simulink model "vuum_wab_4x1_mux"  (R2012b)
settings: Solver=ode45  StartTime=0.0  StopTime=10.0  RelTol=1e-3
libraries: xbsIndex_r4 x210
settings Model: Creator=rng  LastModifiedBy=rng

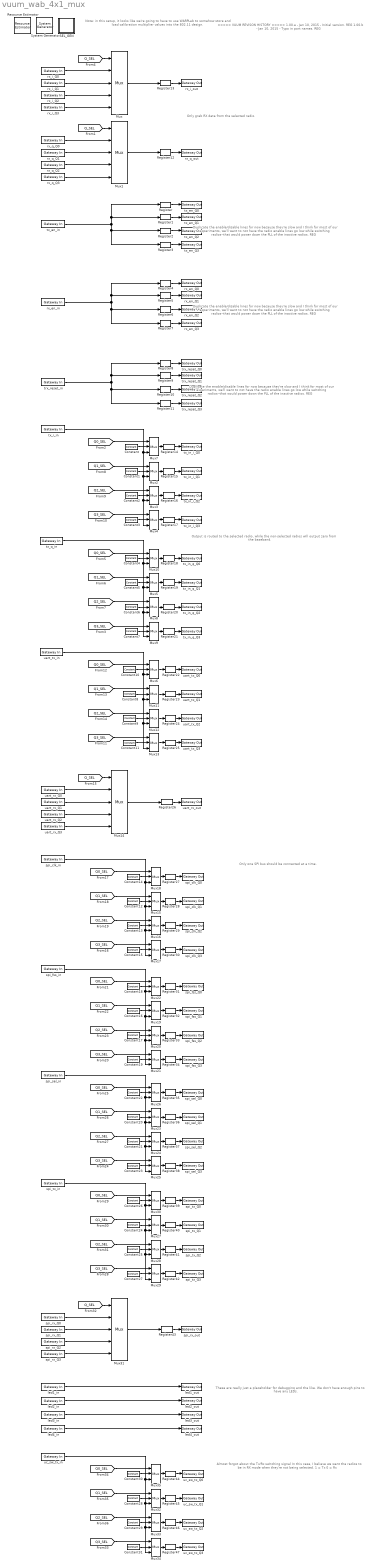
== system vuum_wab_4x1_mux ==
  note: Almost forgot about the Tx/Rx switching signal
      | In this case, I believe we want the radios to be
      | in RX mode when they're not being selected.
      | 1 = Tx
      | 0 = Rx
  note: ===== VUUM REVISON HISTORY =====
      | 1.00.a - Jan 10, 2015 - Initial version. REG
      | 1.00.b - Jan 10, 2015 - Typo in port names. REG
  note: These are really just a placeholder for debugging
      | and the like. We don't have enough pins to have any LEDs.
  note: Only one SPI bus should be connected at a time.
  note: Output is routed to the selected radio, while the
      | non-selected radios will output zero from the
      | baseband.
  note: Duplicate the enable/disable lines for now
      | because they're slow and I think for most
      | of our experiments, we'll want to not have
      | the radio enable lines go low while switching
      | radios--that would power down the PLL of the
      | inactive radios. REG
  note: Only grab RX data from the selected radio.
  note: Note: in this setup, it looks like we're going to have to use WARPLab
      | to somehow store and load calibration multiplier values into the 802.11
      | design.
  note: Duplicate the enable/disable lines for now
      | because they're slow and I think for most
      | of our experiments, we'll want to not have
      | the radio enable lines go low while switching
      | radios--that would power down the PLL of the
      | inactive radios. REG
  note: Duplicate the enable/disable lines for now
      | because they're slow and I think for most
      | of our experiments, we'll want to not have
      | the radio enable lines go low while switching
      | radios--that would power down the PLL of the
      | inactive radios. REG
  " System Generator" : xbsIndex_r4/ System Generator  Tag=genX  xilinxfamily=virtex6  part=xc6vlx240t  speed=-2  package=ff1156  synthesis_tool=XST  clock_wrapper=Clock Enables  directory=./vuum_wab_4x1_mux  proj_type=Project Navigator  Synth_file=XST Defaults  Impl_file=ISE Defaults  testbench=off  simulink_period=1  sysclk_period=10  dcm_input_clock_period=100  incr_netlist=off  trim_vbits=Everywhere in SubSystem  dbl_ovrd=According to Block Masks  core_generation=According to Block Masks  run_coregen=off  deprecated_control=off  eval_field=0  block_type=sysgen
      settings: block_version=10.1.3
  Constant{,1..7} (8 alike) : xbsIndex_r4/Constant  const=0  gui_display_data_type=Fixed-point  arith_type=Signed (2's comp)  n_bits=12  bin_pt=11  preci_type=Single  exp_width=8  frac_width=24  explicit_period=off  period=1  equ=P=C  opselect=C  inp2=PCIN>>17  opr=+  inp1=P  carry=CIN  dbl_ovrd=off  block_type=constant
  Constant{8..31} (24 alike) : xbsIndex_r4/Constant  const=0  gui_display_data_type=Boolean  arith_type=Boolean  n_bits=12  bin_pt=11  preci_type=Single  exp_width=8  frac_width=24  explicit_period=off  period=1  equ=P=C  opselect=C  inp2=PCIN>>17  opr=+  inp1=P  carry=CIN  dbl_ovrd=off  block_type=constant
  Mux{,1,14,31} (4 alike) : xbsIndex_r4/Mux  inputs=4  en=off  latency=0  precision=Full  arith_type=Unsigned  n_bits=16  bin_pt=14  quantization=Truncate  overflow=Wrap  dbl_ovrd=off  block_type=mux
  Mux{2..13,15..30,32..35} (32 alike) : xbsIndex_r4/Mux  inputs=2  en=off  latency=0  precision=Full  arith_type=Unsigned  n_bits=16  bin_pt=14  quantization=Truncate  overflow=Wrap  dbl_ovrd=off  block_type=mux
  Register{,1..47} (48 alike) : xbsIndex_r4/Register  init=0  rst=off  en=off  dbl_ovrd=off  block_type=register
  Resource Estimator : xbsIndex_r4/Resource Estimator  Tag=resEstTag  Slices=3628  FFs=4465  BRAMs=0  LUTs=6136  IOBs=365  EBMs=48  TBUFs=0  xl_use_estimator_area=off  est_options=Post Map  xl_estimator_area=[3628 4465 0 6136 365 48 0]  block_type=resource_estimator
      settings: AttributesFormatString=Resource\nEstimator  block_version=10.1.3
  SEL_GEN : Subsystem
  led1_in : xbsIndex_r4/Gateway In  gui_display_data_type=Boolean  arith_type=Boolean  n_bits=12  bin_pt=11  preci_type=Single  exp_width=8  frac_width=24  quantization="Round  (unbiased: +/- Inf)"  overflow=Saturate  period=1  dbl_ovrd=off  timing_constraint=None  locs_specified=off  LOCs={}  UseAsADC=off  ADCChannel='1'  inherit_from_input=off  hdl_port=on  block_type=gatewayin
  led1_out : xbsIndex_r4/Gateway Out  inherit_from_input=off  hdl_port=on  timing_constraint=None  locs_specified=off  LOCs={}  UseAsDAC=off  DACChannel='1'  block_type=gatewayout
  led2_in : xbsIndex_r4/Gateway In  gui_display_data_type=Boolean  arith_type=Boolean  n_bits=12  bin_pt=11  preci_type=Single  exp_width=8  frac_width=24  quantization="Round  (unbiased: +/- Inf)"  overflow=Saturate  period=1  dbl_ovrd=off  timing_constraint=None  locs_specified=off  LOCs={}  UseAsADC=off  ADCChannel='1'  inherit_from_input=off  hdl_port=on  block_type=gatewayin
  led2_out : xbsIndex_r4/Gateway Out  inherit_from_input=off  hdl_port=on  timing_constraint=None  locs_specified=off  LOCs={}  UseAsDAC=off  DACChannel='1'  block_type=gatewayout
  led3_in : xbsIndex_r4/Gateway In  gui_display_data_type=Boolean  arith_type=Boolean  n_bits=12  bin_pt=11  preci_type=Single  exp_width=8  frac_width=24  quantization="Round  (unbiased: +/- Inf)"  overflow=Saturate  period=1  dbl_ovrd=off  timing_constraint=None  locs_specified=off  LOCs={}  UseAsADC=off  ADCChannel='1'  inherit_from_input=off  hdl_port=on  block_type=gatewayin
  led3_out : xbsIndex_r4/Gateway Out  inherit_from_input=off  hdl_port=on  timing_constraint=None  locs_specified=off  LOCs={}  UseAsDAC=off  DACChannel='1'  block_type=gatewayout
  led4_in : xbsIndex_r4/Gateway In  gui_display_data_type=Boolean  arith_type=Boolean  n_bits=12  bin_pt=11  preci_type=Single  exp_width=8  frac_width=24  quantization="Round  (unbiased: +/- Inf)"  overflow=Saturate  period=1  dbl_ovrd=off  timing_constraint=None  locs_specified=off  LOCs={}  UseAsADC=off  ADCChannel='1'  inherit_from_input=off  hdl_port=on  block_type=gatewayin
  led4_out : xbsIndex_r4/Gateway Out  inherit_from_input=off  hdl_port=on  timing_constraint=None  locs_specified=off  LOCs={}  UseAsDAC=off  DACChannel='1'  block_type=gatewayout
  rx_en_Q{0..3} (4 alike) : xbsIndex_r4/Gateway Out  inherit_from_input=off  hdl_port=on  timing_constraint=None  locs_specified=off  LOCs={}  UseAsDAC=off  DACChannel='1'  block_type=gatewayout
  rx_en_in : xbsIndex_r4/Gateway In  gui_display_data_type=Boolean  arith_type=Boolean  n_bits=12  bin_pt=11  preci_type=Single  exp_width=8  frac_width=24  quantization="Round  (unbiased: +/- Inf)"  overflow=Saturate  period=1  dbl_ovrd=off  timing_constraint=None  locs_specified=off  LOCs={}  UseAsADC=off  ADCChannel='1'  inherit_from_input=off  hdl_port=on  block_type=gatewayin
  rx_i_Q{0..3} (4 alike) : xbsIndex_r4/Gateway In  gui_display_data_type=Fixed-point  arith_type="Signed  (2's comp)"  n_bits=12  bin_pt=11  preci_type=Single  exp_width=8  frac_width=24  quantization="Round  (unbiased: +/- Inf)"  overflow=Saturate  period=1  dbl_ovrd=off  timing_constraint=None  locs_specified=off  LOCs={}  UseAsADC=off  ADCChannel='1'  inherit_from_input=off  hdl_port=on  block_type=gatewayin
  rx_i_out : xbsIndex_r4/Gateway Out  inherit_from_input=off  hdl_port=on  timing_constraint=None  locs_specified=off  LOCs={}  UseAsDAC=off  DACChannel='1'  block_type=gatewayout
  rx_q_Q{0..3} (4 alike) : xbsIndex_r4/Gateway In  gui_display_data_type=Fixed-point  arith_type="Signed  (2's comp)"  n_bits=12  bin_pt=11  preci_type=Single  exp_width=8  frac_width=24  quantization="Round  (unbiased: +/- Inf)"  overflow=Saturate  period=1  dbl_ovrd=off  timing_constraint=None  locs_specified=off  LOCs={}  UseAsADC=off  ADCChannel='1'  inherit_from_input=off  hdl_port=on  block_type=gatewayin
  rx_q_out : xbsIndex_r4/Gateway Out  inherit_from_input=off  hdl_port=on  timing_constraint=None  locs_specified=off  LOCs={}  UseAsDAC=off  DACChannel='1'  block_type=gatewayout
  spi_clk_Q{0..3} (4 alike) : xbsIndex_r4/Gateway Out  inherit_from_input=off  hdl_port=on  timing_constraint=None  locs_specified=off  LOCs={}  UseAsDAC=off  DACChannel='1'  block_type=gatewayout
  spi_clk_in : xbsIndex_r4/Gateway In  gui_display_data_type=Boolean  arith_type=Boolean  n_bits=12  bin_pt=11  preci_type=Single  exp_width=8  frac_width=24  quantization="Round  (unbiased: +/- Inf)"  overflow=Saturate  period=1  dbl_ovrd=off  timing_constraint=None  locs_specified=off  LOCs={}  UseAsADC=off  ADCChannel='1'  inherit_from_input=off  hdl_port=on  block_type=gatewayin
  spi_fss_Q{0..3} (4 alike) : xbsIndex_r4/Gateway Out  inherit_from_input=off  hdl_port=on  timing_constraint=None  locs_specified=off  LOCs={}  UseAsDAC=off  DACChannel='1'  block_type=gatewayout
  spi_fss_in : xbsIndex_r4/Gateway In  gui_display_data_type=Boolean  arith_type=Boolean  n_bits=12  bin_pt=11  preci_type=Single  exp_width=8  frac_width=24  quantization="Round  (unbiased: +/- Inf)"  overflow=Saturate  period=1  dbl_ovrd=off  timing_constraint=None  locs_specified=off  LOCs={}  UseAsADC=off  ADCChannel='1'  inherit_from_input=off  hdl_port=on  block_type=gatewayin
  spi_rx_Q{0..3} (4 alike) : xbsIndex_r4/Gateway In  gui_display_data_type=Boolean  arith_type=Boolean  n_bits=12  bin_pt=11  preci_type=Single  exp_width=8  frac_width=24  quantization="Round  (unbiased: +/- Inf)"  overflow=Saturate  period=1  dbl_ovrd=off  timing_constraint=None  locs_specified=off  LOCs={}  UseAsADC=off  ADCChannel='1'  inherit_from_input=off  hdl_port=on  block_type=gatewayin
  spi_rx_out : xbsIndex_r4/Gateway Out  inherit_from_input=off  hdl_port=on  timing_constraint=None  locs_specified=off  LOCs={}  UseAsDAC=off  DACChannel='1'  block_type=gatewayout
  spi_sel_Q{0..3} (4 alike) : xbsIndex_r4/Gateway Out  inherit_from_input=off  hdl_port=on  timing_constraint=None  locs_specified=off  LOCs={}  UseAsDAC=off  DACChannel='1'  block_type=gatewayout
  spi_sel_in : xbsIndex_r4/Gateway In  gui_display_data_type=Boolean  arith_type=Boolean  n_bits=12  bin_pt=11  preci_type=Single  exp_width=8  frac_width=24  quantization="Round  (unbiased: +/- Inf)"  overflow=Saturate  period=1  dbl_ovrd=off  timing_constraint=None  locs_specified=off  LOCs={}  UseAsADC=off  ADCChannel='1'  inherit_from_input=off  hdl_port=on  block_type=gatewayin
  spi_tx_Q{0..3} (4 alike) : xbsIndex_r4/Gateway Out  inherit_from_input=off  hdl_port=on  timing_constraint=None  locs_specified=off  LOCs={}  UseAsDAC=off  DACChannel='1'  block_type=gatewayout
  spi_tx_in : xbsIndex_r4/Gateway In  gui_display_data_type=Boolean  arith_type=Boolean  n_bits=12  bin_pt=11  preci_type=Single  exp_width=8  frac_width=24  quantization="Round  (unbiased: +/- Inf)"  overflow=Saturate  period=1  dbl_ovrd=off  timing_constraint=None  locs_specified=off  LOCs={}  UseAsADC=off  ADCChannel='1'  inherit_from_input=off  hdl_port=on  block_type=gatewayin
  trx_reset_Q{0..3} (4 alike) : xbsIndex_r4/Gateway Out  inherit_from_input=off  hdl_port=on  timing_constraint=None  locs_specified=off  LOCs={}  UseAsDAC=off  DACChannel='1'  block_type=gatewayout
  trx_reset_in : xbsIndex_r4/Gateway In  gui_display_data_type=Boolean  arith_type=Boolean  n_bits=12  bin_pt=11  preci_type=Single  exp_width=8  frac_width=24  quantization="Round  (unbiased: +/- Inf)"  overflow=Saturate  period=1  dbl_ovrd=off  timing_constraint=None  locs_specified=off  LOCs={}  UseAsADC=off  ADCChannel='1'  inherit_from_input=off  hdl_port=on  block_type=gatewayin
  tx_en_Q{0..3} (4 alike) : xbsIndex_r4/Gateway Out  inherit_from_input=off  hdl_port=on  timing_constraint=None  locs_specified=off  LOCs={}  UseAsDAC=off  DACChannel='1'  block_type=gatewayout
  tx_en_in : xbsIndex_r4/Gateway In  gui_display_data_type=Boolean  arith_type=Boolean  n_bits=12  bin_pt=11  preci_type=Single  exp_width=8  frac_width=24  quantization="Round  (unbiased: +/- Inf)"  overflow=Saturate  period=1  dbl_ovrd=off  timing_constraint=None  locs_specified=off  LOCs={}  UseAsADC=off  ADCChannel='1'  inherit_from_input=off  hdl_port=on  block_type=gatewayin
  tx_i_in : xbsIndex_r4/Gateway In  gui_display_data_type=Fixed-point  arith_type="Signed  (2's comp)"  n_bits=12  bin_pt=11  preci_type=Single  exp_width=8  frac_width=24  quantization="Round  (unbiased: +/- Inf)"  overflow=Saturate  period=1  dbl_ovrd=off  timing_constraint=None  locs_specified=off  LOCs={}  UseAsADC=off  ADCChannel='1'  inherit_from_input=off  hdl_port=on  block_type=gatewayin
  tx_in_i_Q{0..3} (4 alike) : xbsIndex_r4/Gateway Out  inherit_from_input=off  hdl_port=on  timing_constraint=None  locs_specified=off  LOCs={}  UseAsDAC=off  DACChannel='1'  block_type=gatewayout
  tx_in_q_Q{0..3} (4 alike) : xbsIndex_r4/Gateway Out  inherit_from_input=off  hdl_port=on  timing_constraint=None  locs_specified=off  LOCs={}  UseAsDAC=off  DACChannel='1'  block_type=gatewayout
  tx_q_in : xbsIndex_r4/Gateway In  gui_display_data_type=Fixed-point  arith_type="Signed  (2's comp)"  n_bits=12  bin_pt=11  preci_type=Single  exp_width=8  frac_width=24  quantization="Round  (unbiased: +/- Inf)"  overflow=Saturate  period=1  dbl_ovrd=off  timing_constraint=None  locs_specified=off  LOCs={}  UseAsADC=off  ADCChannel='1'  inherit_from_input=off  hdl_port=on  block_type=gatewayin
  uart_rx_Q{0..3} (4 alike) : xbsIndex_r4/Gateway In  gui_display_data_type=Boolean  arith_type=Boolean  n_bits=12  bin_pt=11  preci_type=Single  exp_width=8  frac_width=24  quantization="Round  (unbiased: +/- Inf)"  overflow=Saturate  period=1  dbl_ovrd=off  timing_constraint=None  locs_specified=off  LOCs={}  UseAsADC=off  ADCChannel='1'  inherit_from_input=off  hdl_port=on  block_type=gatewayin
  uart_rx_out : xbsIndex_r4/Gateway Out  inherit_from_input=off  hdl_port=on  timing_constraint=None  locs_specified=off  LOCs={}  UseAsDAC=off  DACChannel='1'  block_type=gatewayout
  uart_tx_Q{0..3} (4 alike) : xbsIndex_r4/Gateway Out  inherit_from_input=off  hdl_port=on  timing_constraint=None  locs_specified=off  LOCs={}  UseAsDAC=off  DACChannel='1'  block_type=gatewayout
  uart_tx_in : xbsIndex_r4/Gateway In  gui_display_data_type=Boolean  arith_type=Boolean  n_bits=12  bin_pt=11  preci_type=Single  exp_width=8  frac_width=24  quantization="Round  (unbiased: +/- Inf)"  overflow=Saturate  period=1  dbl_ovrd=off  timing_constraint=None  locs_specified=off  LOCs={}  UseAsADC=off  ADCChannel='1'  inherit_from_input=off  hdl_port=on  block_type=gatewayin
  uc_sw_tx_Q{0..3} (4 alike) : xbsIndex_r4/Gateway Out  inherit_from_input=off  hdl_port=on  timing_constraint=None  locs_specified=off  LOCs={}  UseAsDAC=off  DACChannel='1'  block_type=gatewayout
  uc_sw_tx_in : xbsIndex_r4/Gateway In  gui_display_data_type=Boolean  arith_type=Boolean  n_bits=12  bin_pt=11  preci_type=Single  exp_width=8  frac_width=24  quantization="Round  (unbiased: +/- Inf)"  overflow=Saturate  period=1  dbl_ovrd=off  timing_constraint=None  locs_specified=off  LOCs={}  UseAsADC=off  ADCChannel='1'  inherit_from_input=off  hdl_port=on  block_type=gatewayin
  wires:
  [Q_SEL] -> Mux/1
  rx_i_Q0/1 -> Mux/2
  rx_i_Q1/1 -> Mux/3
  rx_i_Q2/1 -> Mux/4
  rx_i_Q3/1 -> Mux/5
  [Q_SEL] -> Mux1/1
  rx_q_Q0/1 -> Mux1/2
  rx_q_Q1/1 -> Mux1/3
  rx_q_Q2/1 -> Mux1/4
  rx_q_Q3/1 -> Mux1/5
  Mux/1 -> Register13/1
  Mux1/1 -> Register12/1
  tx_en_in/1 -> Register2/1, Register3/1, Register1/1, Register/1
  Register/1 -> tx_en_Q0/1
  Register1/1 -> tx_en_Q1/1
  Register2/1 -> tx_en_Q2/1
  Register3/1 -> tx_en_Q3/1
  rx_en_in/1 -> Register6/1, Register7/1, Register5/1, Register4/1
  Register4/1 -> rx_en_Q0/1
  Register5/1 -> rx_en_Q1/1
  Register6/1 -> rx_en_Q2/1
  Register7/1 -> rx_en_Q3/1
  trx_reset_in/1 -> Register10/1, Register11/1, Register9/1, Register8/1
  Register8/1 -> trx_reset_Q0/1
  Register9/1 -> trx_reset_Q1/1
  Register10/1 -> trx_reset_Q2/1
  Register11/1 -> trx_reset_Q3/1
  Constant/1 -> Mux7/2
  [Q0_SEL] -> Mux7/1
  tx_i_in/1 -> Mux4/3, Mux3/3, Mux2/3, Mux7/3
  Constant1/1 -> Mux2/2
  [Q1_SEL] -> Mux2/1
  Constant2/1 -> Mux3/2
  [Q2_SEL] -> Mux3/1
  Constant3/1 -> Mux4/2
  [Q3_SEL] -> Mux4/1
  Constant4/1 -> Mux10/2
  [Q0_SEL] -> Mux10/1
  tx_q_in/1 -> Mux9/3, Mux8/3, Mux5/3, Mux10/3
  Constant5/1 -> Mux5/2
  [Q1_SEL] -> Mux5/1
  Constant6/1 -> Mux8/2
  [Q2_SEL] -> Mux8/1
  Constant7/1 -> Mux9/2
  [Q3_SEL] -> Mux9/1
  Constant10/1 -> Mux6/2
  [Q0_SEL] -> Mux6/1
  uart_tx_in/1 -> Mux13/3, Mux12/3, Mux11/3, Mux6/3
  Constant8/1 -> Mux11/2
  [Q1_SEL] -> Mux11/1
  Constant9/1 -> Mux12/2
  [Q2_SEL] -> Mux12/1
  Constant11/1 -> Mux13/2
  [Q3_SEL] -> Mux13/1
  [Q_SEL] -> Mux14/1
  uart_rx_Q0/1 -> Mux14/2
  uart_rx_Q1/1 -> Mux14/3
  uart_rx_Q2/1 -> Mux14/4
  uart_rx_Q3/1 -> Mux14/5
  Mux14/1 -> Register26/1
  Constant14/1 -> Mux18/2
  [Q0_SEL] -> Mux18/1
  spi_clk_in/1 -> Mux17/3, Mux16/3, Mux15/3, Mux18/3
  Constant12/1 -> Mux15/2
  [Q1_SEL] -> Mux15/1
  Constant13/1 -> Mux16/2
  [Q2_SEL] -> Mux16/1
  Constant15/1 -> Mux17/2
  [Q3_SEL] -> Mux17/1
  Constant18/1 -> Mux22/2
  [Q0_SEL] -> Mux22/1
  spi_fss_in/1 -> Mux21/3, Mux20/3, Mux19/3, Mux22/3
  Constant16/1 -> Mux19/2
  [Q1_SEL] -> Mux19/1
  Constant17/1 -> Mux20/2
  [Q2_SEL] -> Mux20/1
  Constant19/1 -> Mux21/2
  [Q3_SEL] -> Mux21/1
  Constant22/1 -> Mux26/2
  [Q0_SEL] -> Mux26/1
  spi_sel_in/1 -> Mux25/3, Mux24/3, Mux23/3, Mux26/3
  Constant20/1 -> Mux23/2
  [Q1_SEL] -> Mux23/1
  Constant21/1 -> Mux24/2
  [Q2_SEL] -> Mux24/1
  Constant23/1 -> Mux25/2
  [Q3_SEL] -> Mux25/1
  Constant26/1 -> Mux30/2
  [Q0_SEL] -> Mux30/1
  spi_tx_in/1 -> Mux29/3, Mux28/3, Mux27/3, Mux30/3
  Constant24/1 -> Mux27/2
  [Q1_SEL] -> Mux27/1
  [Q2_SEL] -> Mux28/1
  [Q3_SEL] -> Mux29/1
  Register12/1 -> rx_q_out/1
  Register13/1 -> rx_i_out/1
  Mux7/1 -> Register14/1
  Register14/1 -> tx_in_i_Q0/1
  Mux2/1 -> Register15/1
  Register15/1 -> tx_in_i_Q1/1
  Mux3/1 -> Register16/1
  Register16/1 -> tx_in_i_Q2/1
  Mux4/1 -> Register17/1
  Register17/1 -> tx_in_i_Q3/1
  Register18/1 -> tx_in_q_Q0/1
  Register19/1 -> tx_in_q_Q1/1
  Register20/1 -> tx_in_q_Q2/1
  Register21/1 -> tx_in_q_Q3/1
  Mux10/1 -> Register18/1
  Mux5/1 -> Register19/1
  Mux8/1 -> Register20/1
  Mux9/1 -> Register21/1
  Register22/1 -> uart_tx_Q0/1
  Register23/1 -> uart_tx_Q1/1
  Register24/1 -> uart_tx_Q2/1
  Register25/1 -> uart_tx_Q3/1
  Mux6/1 -> Register22/1
  Mux11/1 -> Register23/1
  Mux12/1 -> Register24/1
  Mux13/1 -> Register25/1
  Register26/1 -> uart_rx_out/1
  Mux18/1 -> Register27/1
  Register27/1 -> spi_clk_Q0/1
  Mux15/1 -> Register28/1
  Register28/1 -> spi_clk_Q1/1
  Mux16/1 -> Register29/1
  Register29/1 -> spi_clk_Q2/1
  Mux17/1 -> Register30/1
  Register30/1 -> spi_clk_Q3/1
  Register31/1 -> spi_fss_Q0/1
  Register32/1 -> spi_fss_Q1/1
  Register33/1 -> spi_fss_Q2/1
  Register34/1 -> spi_fss_Q3/1
  Mux22/1 -> Register31/1
  Mux19/1 -> Register32/1
  Mux20/1 -> Register33/1
  Mux21/1 -> Register34/1
  Register35/1 -> spi_sel_Q0/1
  Register36/1 -> spi_sel_Q1/1
  Register37/1 -> spi_sel_Q2/1
  Register38/1 -> spi_sel_Q3/1
  Mux26/1 -> Register35/1
  Mux23/1 -> Register36/1
  Mux24/1 -> Register37/1
  Mux25/1 -> Register38/1
  Register39/1 -> spi_tx_Q0/1
  Register40/1 -> spi_tx_Q1/1
  Register41/1 -> spi_tx_Q2/1
  Register42/1 -> spi_tx_Q3/1
  Mux30/1 -> Register39/1
  Mux27/1 -> Register40/1
  Mux28/1 -> Register41/1
  Mux29/1 -> Register42/1
  [Q_SEL] -> Mux31/1
  spi_rx_Q0/1 -> Mux31/2
  spi_rx_Q1/1 -> Mux31/3
  spi_rx_Q2/1 -> Mux31/4
  spi_rx_Q3/1 -> Mux31/5
  Mux31/1 -> Register43/1
  Register43/1 -> spi_rx_out/1
  led1_in/1 -> led1_out/1
  led2_in/1 -> led2_out/1
  led3_in/1 -> led3_out/1
  led4_in/1 -> led4_out/1
  Constant27/1 -> Mux29/2
  Constant25/1 -> Mux28/2
  Constant30/1 -> Mux35/2
  [Q0_SEL] -> Mux35/1
  uc_sw_tx_in/1 -> Mux34/3, Mux33/3, Mux32/3, Mux35/3
  Constant28/1 -> Mux32/2
  [Q1_SEL] -> Mux32/1
  Constant29/1 -> Mux33/2
  [Q2_SEL] -> Mux33/1
  Constant31/1 -> Mux34/2
  [Q3_SEL] -> Mux34/1
  Register44/1 -> uc_sw_tx_Q0/1
  Register45/1 -> uc_sw_tx_Q1/1
  Register46/1 -> uc_sw_tx_Q2/1
  Register47/1 -> uc_sw_tx_Q3/1
  Mux35/1 -> Register44/1
  Mux32/1 -> Register45/1
  Mux33/1 -> Register46/1
  Mux34/1 -> Register47/1

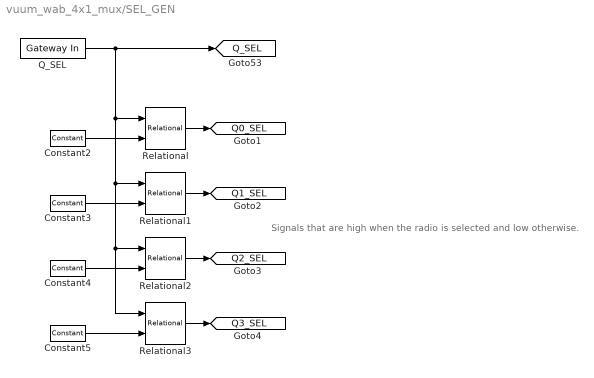
== system vuum_wab_4x1_mux/SEL_GEN ==
  note: Signals that are high when the
      | radio is selected and low otherwise.
  Constant2 : xbsIndex_r4/Constant  const=0  gui_display_data_type=Fixed-point  arith_type=Unsigned  n_bits=2  bin_pt=0  preci_type=Single  exp_width=8  frac_width=24  explicit_period=off  period=1  equ=P=C  opselect=C  inp2=PCIN>>17  opr=+  inp1=P  carry=CIN  dbl_ovrd=off  block_type=constant
  Constant3 : xbsIndex_r4/Constant  const=1  gui_display_data_type=Fixed-point  arith_type=Unsigned  n_bits=2  bin_pt=0  preci_type=Single  exp_width=8  frac_width=24  explicit_period=off  period=1  equ=P=C  opselect=C  inp2=PCIN>>17  opr=+  inp1=P  carry=CIN  dbl_ovrd=off  block_type=constant
  Constant4 : xbsIndex_r4/Constant  const=2  gui_display_data_type=Fixed-point  arith_type=Unsigned  n_bits=2  bin_pt=0  preci_type=Single  exp_width=8  frac_width=24  explicit_period=off  period=1  equ=P=C  opselect=C  inp2=PCIN>>17  opr=+  inp1=P  carry=CIN  dbl_ovrd=off  block_type=constant
  Constant5 : xbsIndex_r4/Constant  const=3  gui_display_data_type=Fixed-point  arith_type=Unsigned  n_bits=2  bin_pt=0  preci_type=Single  exp_width=8  frac_width=24  explicit_period=off  period=1  equ=P=C  opselect=C  inp2=PCIN>>17  opr=+  inp1=P  carry=CIN  dbl_ovrd=off  block_type=constant
  Q_SEL : xbsIndex_r4/Gateway In  gui_display_data_type=Fixed-point  arith_type=Unsigned  n_bits=2  bin_pt=0  preci_type=Single  exp_width=8  frac_width=24  quantization="Round  (unbiased: +/- Inf)"  overflow=Saturate  period=1  dbl_ovrd=off  timing_constraint=None  locs_specified=off  LOCs={}  UseAsADC=off  ADCChannel='1'  inherit_from_input=off  hdl_port=on  block_type=gatewayin
  Relational{,1..3} (4 alike) : xbsIndex_r4/Relational  mode=a=b  en=off  latency=0  dbl_ovrd=off  block_type=relational
  tag scope: Q0_SEL=global, Q1_SEL=global, Q2_SEL=global, Q3_SEL=global, Q_SEL=global
  wires:
  Constant5/1 -> Relational3/2
  Constant2/1 -> Relational/2
  Q_SEL/1 -> Relational3/1, Relational2/1, Relational1/1, Relational/1, [Q_SEL]
  Constant4/1 -> Relational2/2
  Constant3/1 -> Relational1/2
  Relational1/1 -> [Q1_SEL]
  Relational3/1 -> [Q3_SEL]
  Relational2/1 -> [Q2_SEL]
  Relational/1 -> [Q0_SEL]
